simulink model "Tutorial2_ModelBlocks"  (Simulink 9.1)
settings: Solver=FixedStepAuto  StartTime=0.0  StopTime=10.0  RelTol=1e-3
libraries: WBToolboxLibrary x4
settings Model: SuppressorTable=22 serialization::archive 11 0 6 0 0 0 1 0  Creator=dferigo  LastModifiedBy=dferigo
settings DataIOCC: SaveFormat=Dataset
settings OptimizationCC: LifeSpan=auto
settings DebuggingCC: UnderspecifiedInitializationDetection=Simplified  MergeDetectMultiDrivingBlocksExec=error  SFUnexpectedBacktrackingDiag=error  SFNoUnconditionalDefaultTransitionDiag=error  SFExecutionAtInitializationDiag=warning
settings HardwareCC: ProdBitPerPointer=64  ProdBitPerSizeT=64  ProdBitPerPtrDiffT=64  ProdLargestAtomicFloat=Float  ProdIntDivRoundTo=Zero  ProdEndianess=LittleEndian  ProdWordSize=64  ProdHWDeviceType=Intel->x86-64 (Windows64)
settings ModelReferenceCC: PropagateSignalLabelsOutOfModel=on
settings CodeAppCC: StateflowObjectComments=off
settings GRTTargetCC: TargetLangStandard=C99 (ISO)  CombineOutputUpdateFcns=on  GRTInterface=off
settings ConfigComp: CovMetricSettings=dwe  CovHtmlReporting=off  CovSaveCumulativeToWorkspaceVar=off  CovSaveSingleToWorkspaceVar=off  CovExternalEMLEnable=on

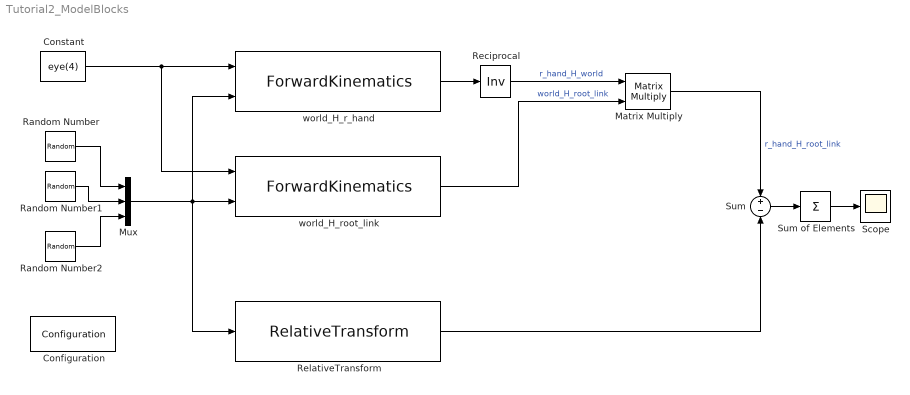
== system Tutorial2_ModelBlocks ==
  Configuration : WBToolboxLibrary/Utilities/Configuration  ConfigSource=Mask  ConfigObject='WBTConfigRobot'  RobotName='doesnotmatter'  UrdfFile='model.urdf'  ControlledJoints={'r_elbow','r_shoulder_pitch','torso_roll'}  ControlBoardsNames={'doesnotmatter'}  LocalName='doesnotmatter'  GravityVector=[0,0,-9.81]
      settings: SourceProductName=WholeBodyToolbox
  Constant : Constant  Value=eye(4)
  Matrix Multiply : Product  Multiplication=Matrix(*)
  Mux : Mux  Inputs=3
  Random Number : RandomNumber  Variance=20 / 180 * pi  SampleTime=0.1
  Random Number1 : RandomNumber  Variance=20 / 180 * pi  SampleTime=0.1
  Random Number2 : RandomNumber  Variance=20 / 180 * pi  SampleTime=0.1
  Reciprocal : Product  Inputs=/  Multiplication=Matrix(*)
  RelativeTransform : WBToolboxLibrary/Model/Kinematics/RelativeTransform  frame1='r_hand'  frame2='root_link'
      settings: SourceProductName=WholeBodyToolbox
  Scope : Scope
  Sum : Sum  Inputs=+|-
  Sum of Elements : Sum  Inputs=+
  world_H_r_hand : WBToolboxLibrary/Model/Kinematics/ForwardKinematics  frameName='r_hand'
      settings: SourceProductName=WholeBodyToolbox
  world_H_root_link : WBToolboxLibrary/Model/Kinematics/ForwardKinematics  frameName='root_link'
      settings: SourceProductName=WholeBodyToolbox
  wires:
  Constant/1 -> world_H_root_link/1, world_H_r_hand/1
  world_H_r_hand/1 -> Reciprocal/1
  Reciprocal/1 -> Matrix Multiply/1  "r_hand_H_world"
  world_H_root_link/1 -> Matrix Multiply/2  "world_H_root_link"
  Matrix Multiply/1 -> Sum/1  "r_hand_H_root_link"
  RelativeTransform/1 -> Sum/2
  Sum/1 -> Sum of Elements/1
  Mux/1 -> world_H_r_hand/2, world_H_root_link/2, RelativeTransform/1
  Sum of Elements/1 -> Scope/1
  Random Number1/1 -> Mux/2
  Random Number/1 -> Mux/1
  Random Number2/1 -> Mux/3
